simulink model "Em_Project_Fuzzy"  (R2023b)
settings: Solver=VariableStepAuto  StartTime=0.0  StopTime=5  RelTol=1e-3
undefined symbols (not defined in the file): B, J
libraries: fuzblock x1
settings Model: Creator=KEERTHI  LastModifiedBy=KEERTHI

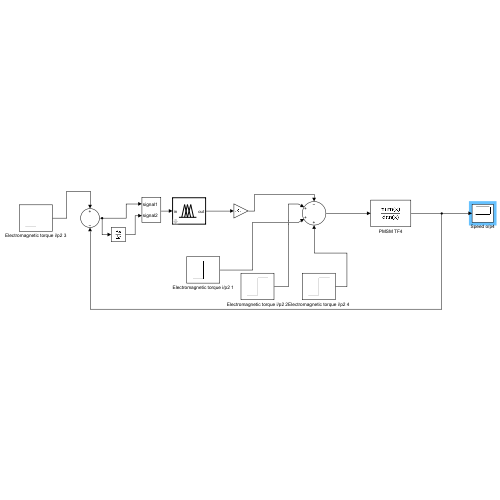
[thumbnail: Simulink's stored preview of the top-level diagram]
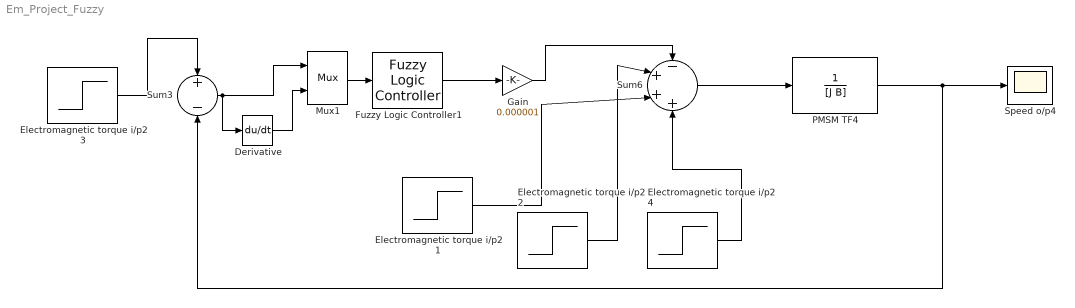
== system Em_Project_Fuzzy ==
  Derivative : Derivative
  Electromagnetic torque i/p2 1 : Step  Time=0.2  After=2  SampleTime=0
  Electromagnetic torque i/p2 2 : Step  Time=0.4  After=3  SampleTime=0
  Electromagnetic torque i/p2 3 : Step  Time=0  After=10  SampleTime=0
  Electromagnetic torque i/p2 4 : Step  Time=0.6  After=4  SampleTime=0
  Fuzzy Logic Controller1 : fuzblock/Fuzzy Logic  Controller  FIS='PMSM_fuzzy_controller.fis'  OutputSampleNumber=101  DataType=double  FuzzifiedInputs=off  RuleFiringStrengths=off  RuleOutputs=off  AggregatedOutputs=off  SimulateUsing=Interpreted execution  OutOfRangeInputValueMessage=warning  NoRuleFiredMessage=warning  EmptyOutputFuzzySetMessage=warning
  Gain : Gain  Gain=0.000001
  Mux1 : Mux  Inputs=2
      settings: DisplayOption=signals
  PMSM TF4 : TransferFcn  Denominator=[J B]
  Speed o/p4 : Scope
  Sum3 : Sum  Inputs=+-
  Sum6 : Sum  Inputs=-+++
  wires:
  Sum3/1 -> Mux1/1, Derivative/1
  PMSM TF4/1 -> Speed o/p4/1, Sum3/2
  Sum6/1 -> PMSM TF4/1
  Mux1/1 -> Fuzzy Logic Controller1/1
  Electromagnetic torque i/p2 3/1 -> Sum3/1
  Derivative/1 -> Mux1/2
  Fuzzy Logic Controller1/1 -> Gain/1
  Gain/1 -> Sum6/1
  Electromagnetic torque i/p2 2/1 -> Sum6/2
  Electromagnetic torque i/p2 1/1 -> Sum6/3
  Electromagnetic torque i/p2 4/1 -> Sum6/4
